simulink model "asyncSAR"  (R2024a)
settings: Solver=VariableStepAuto  StartTime=0.0  StopTime=0.0001844  RelTol=1e-3
model workspace (MAT data in the model file):
  Delay_106 = [1.91e-08 1.91e-08 1.91e-08]
  ENOB_106 = 9.63665810786
  FUNDF_106 = [9716803.44087 10062680.9808]
  FUNDX_106 = [81.3083483231 5.0894765013]
  IMODF_106 = [9396360.87497 10437767.0357]
  IMODX_106 = [6.9941846041 -2.14386455151]
  NoiseFloor_106 = -8.45635788485
  OIP3_106 = 63.5857886051
  SFDR_106 = 76.5977909113
  SINAD_106 = 59.7726818093
  SNR_106 = 59.7770481612
  THD_106 = -82.4847133329
  delay_106 = [1.91e-08 1.91e-08 1.91e-08]
libraries: msbAdcMeasurements x1, spsEdgeDetectorLib x1, dspsigops x1
settings Model: Creator=sjtu  LastModifiedBy=sjtu
settings DebuggingCC: SFUnexpectedBacktrackingDiag=warning

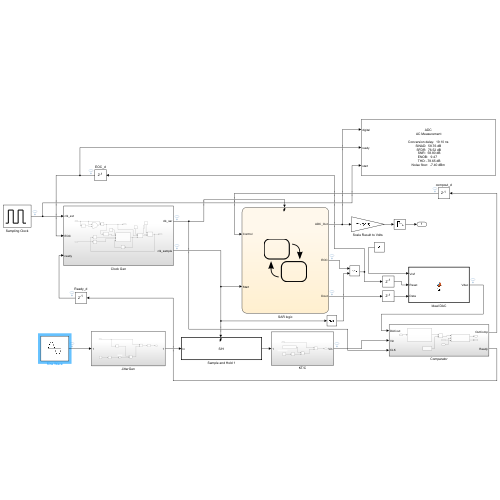
[thumbnail: Simulink's stored preview of the top-level diagram]
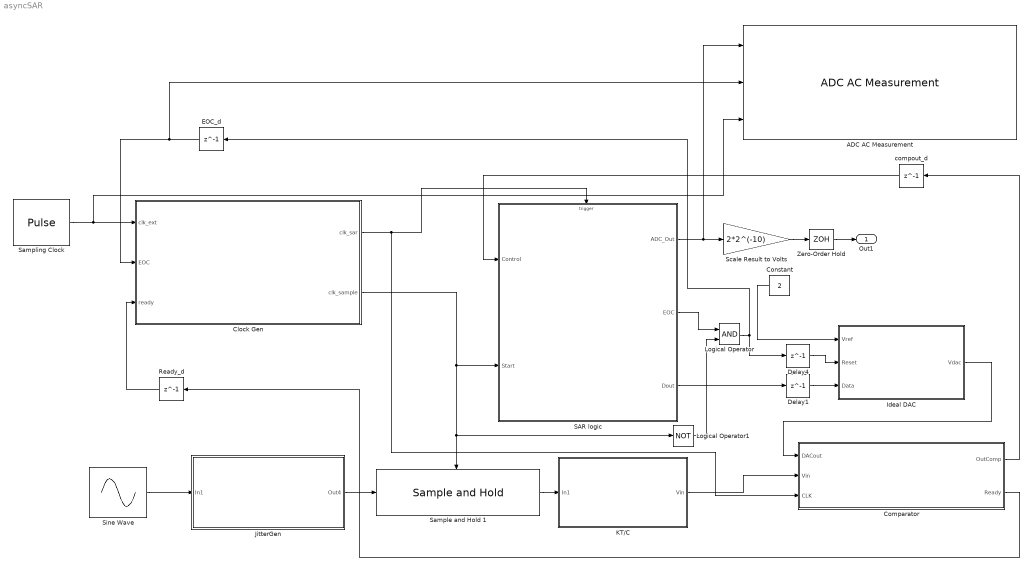
== system asyncSAR ==
  ADC AC Measurement : msbAdcMeasurements/ADC AC Measurement  DistortionMeasurement=Harmonic  InputFrequency=9.729e6  Method=Filter bank (slower, more precise, low leakage)  RBW=48828.125  AutoSetRBW=on  NBits=5  Frequency=5e7  HoldOffTime=0  OutputToWorkspace=off  VariableName=adc_ac_out  ShowSpectrum=off
  Clock Gen : Subsystem
  Comparator : Subsystem
  Constant : Constant  Value=2
  Delay1 : Delay  DelayLength=1  InitialCondition=0  SampleTime=1e-10
  Delay4 : Delay  DelayLength=1  InitialCondition=0  SampleTime=1e-10
  EOC_d : Delay  DelayLength=1  InitialCondition=0  SampleTime=1e-10
  Ideal DAC : MATLAB Function  TreatAsAtomicUnit=on
  JitterGen : Subsystem
  KT/C : Subsystem
  Logical Operator : Logic  AllPortsSameDT=off  OutDataTypeStr=boolean
  Logical Operator1 : Logic  Operator=NOT  AllPortsSameDT=off  OutDataTypeStr=boolean
  Ready_d : Delay  DelayLength=1  InitialCondition=0  SampleTime=1e-10
  SAR logic : Stateflow chart  TreatAsAtomicUnit=on
  Sample and Hold 1 : dspsigops/Sample and Hold  trig=Rising edge  initCond=0  latchinput=off
  Sampling Clock : DiscretePulseGenerator  PulseType=Time based  Period=1/(5e7)  PulseWidth=50  PhaseDelay=1e-9
  Scale Result to Volts : Gain  Gain=2*2^(-10)  ParamDataTypeStr=double  OutDataTypeStr=double
  Sine Wave : Sin  Frequency=2*pi*9.729e6  SampleTime=0
  Zero-Order Hold : ZeroOrderHold  SampleTime=-1
  compout_d : Delay  DelayLength=1  InitialCondition=0  SampleTime=1e-10
  Out1 : Outport
  wires:
  SAR logic/3(Dout) -> Delay1/1
  Delay1/1 -> Ideal DAC/3(Data)
  Zero-Order Hold/1 -> Out1/1
  Constant/1 -> Ideal DAC/1(Vref)
  Ideal DAC/1(Vdac) -> Comparator/1(DACout)
  SAR logic/1(ADC_Out) -> ADC AC Measurement/1, Scale Result to Volts/1
  JitterGen/1(Out4) -> Sample and Hold 1/1
  Scale Result to Volts/1 -> Zero-Order Hold/1
  Sample and Hold 1/1 -> KT/C/1(In1)
  KT/C/1(Vin) -> Comparator/2(Vin)
  Sine Wave/1 -> JitterGen/1(In1)
  Sampling Clock/1 -> ADC AC Measurement/3, Clock Gen/1(clk_ext)
  Comparator/2(Ready) -> Ready_d/1
  Ready_d/1 -> Clock Gen/3(ready)
  EOC_d/1 -> ADC AC Measurement/2, Clock Gen/2(EOC)
  Clock Gen/2(clk_sample) -> SAR logic/2(Start), Sample and Hold 1/Trigger, Logical Operator1/1
  Clock Gen/1(clk_sar) -> Comparator/3(CLK), SAR logic/Trigger
  Delay4/1 -> Ideal DAC/2(Reset)
  Logical Operator1/1 -> Logical Operator/2
  SAR logic/2(EOC) -> Logical Operator/1
  Logical Operator/1 -> EOC_d/1, Delay4/1
  Comparator/1(OutComp) -> compout_d/1
  compout_d/1 -> SAR logic/1(Control)

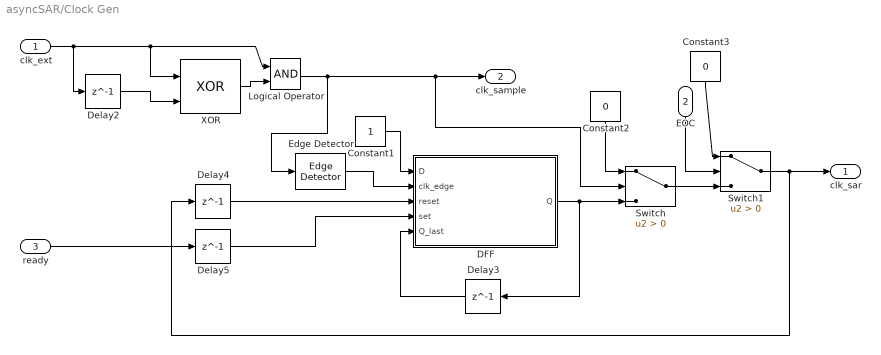
== system asyncSAR/Clock Gen ==
  clk_ext : Inport
  EOC : Inport  Port=2
  ready : Inport  Port=3
  Constant1 : Constant
  Constant2 : Constant  Value=0
  Constant3 : Constant  Value=0
  DFF : MATLAB Function  TreatAsAtomicUnit=on
  Delay2 : Delay  DelayLength=1  InitialCondition=0  SampleTime=2e-9
  Delay3 : Delay  DelayLength=1  InitialCondition=0  SampleTime=1e-10
  Delay4 : Delay  DelayLength=1  InitialCondition=0  SampleTime=4e-10
  Delay5 : Delay  DelayLength=1  InitialCondition=0  SampleTime=4e-10
  Edge Detector : spsEdgeDetectorLib/Edge Detector  model=Rising  ic=0  Ts=0
      settings: LibrarySourceBlock=sps_lib/Control/Edge Detector
  Logical Operator : Logic  AllPortsSameDT=off  OutDataTypeStr=boolean
  Switch : Switch  Criteria=u2 > Threshold  SaturateOnIntegerOverflow=off  InputSameDT=off
  Switch1 : Switch  Criteria=u2 > Threshold  SaturateOnIntegerOverflow=off  InputSameDT=off
  XOR : Logic  Operator=XOR  IconShape=distinctive  AllPortsSameDT=off  OutDataTypeStr=boolean
  clk_sar : Outport
  clk_sample : Outport  Port=2
  wires:
  Delay2/1 -> XOR/2
  clk_ext/1 -> Delay2/1, Logical Operator/1, XOR/1
  Switch/1 -> Switch1/3
  XOR/1 -> Logical Operator/2
  EOC/1 -> Switch1/2
  Logical Operator/1 -> Edge Detector/1, clk_sample/1, Switch/2
  DFF/1(Q) -> Switch/3, Delay3/1
  Constant3/1 -> Switch1/1
  Constant1/1 -> DFF/1(D)
  Delay5/1 -> DFF/4(set)
  Delay3/1 -> DFF/5(Q_last)
  Switch1/1 -> clk_sar/1, Delay4/1
  ready/1 -> Delay5/1
  Delay4/1 -> DFF/3(reset)
  Constant2/1 -> Switch/1
  Edge Detector/1 -> DFF/2(clk_edge)

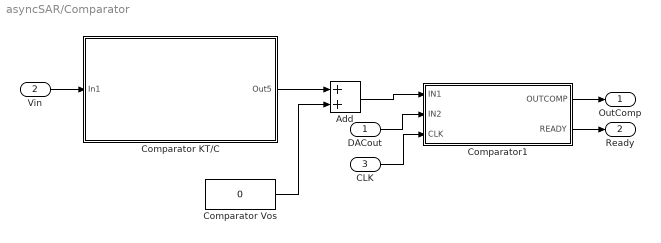
== system asyncSAR/Comparator ==
  DACout : Inport
  Vin : Inport  Port=2
  CLK : Inport  Port=3
  Add : Sum
  Comparator KT/C : Subsystem
  Comparator Vos : Constant  Value=0
  Comparator1 : MATLAB Function  TreatAsAtomicUnit=on
  OutComp : Outport
  Ready : Outport  Port=2
  wires:
  Comparator1/1(OUTCOMP) -> OutComp/1
  Vin/1 -> Comparator KT/C/1(In1)
  Comparator KT/C/1(Out5) -> Add/1
  Add/1 -> Comparator1/1(IN1)
  Comparator Vos/1 -> Add/2
  DACout/1 -> Comparator1/2(IN2)
  CLK/1 -> Comparator1/3(CLK)
  Comparator1/2(READY) -> Ready/1

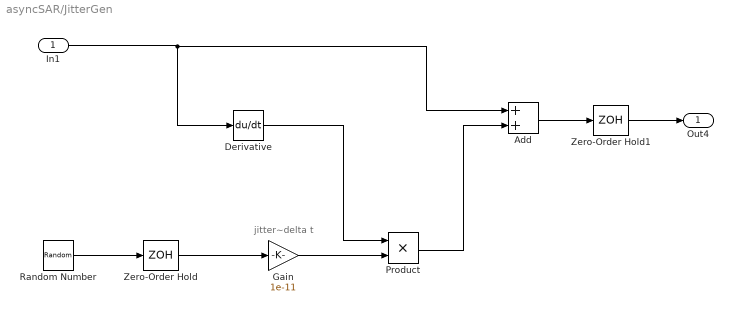
== system asyncSAR/JitterGen ==
  note: jitter~delta t
  In1 : Inport
  Add : Sum
  Derivative : Derivative
  Gain : Gain  Gain=1e-11
  Product : Product
  Random Number : RandomNumber  SampleTime=1e-9
  Zero-Order Hold : ZeroOrderHold  SampleTime=-1
  Zero-Order Hold1 : ZeroOrderHold  SampleTime=-1
  Out4 : Outport
  wires:
  Gain/1 -> Product/2
  Random Number/1 -> Zero-Order Hold/1
  Product/1 -> Add/2
  In1/1 -> Add/1, Derivative/1
  Zero-Order Hold/1 -> Gain/1
  Add/1 -> Zero-Order Hold1/1
  Derivative/1 -> Product/1
  Zero-Order Hold1/1 -> Out4/1

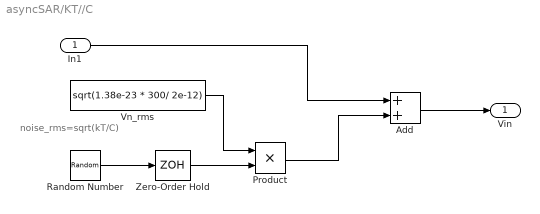
== system asyncSAR/KT//C ==
  note: noise_rms=sqrt(kT/C)
  In1 : Inport
  Add : Sum
  Product : Product
  Random Number : RandomNumber  SampleTime=1e-9
  Vn_rms : Constant  Value=sqrt(1.38e-23 * 300/ 2e-12)
  Zero-Order Hold : ZeroOrderHold  SampleTime=-1
  Vin : Outport
  wires:
  Vn_rms/1 -> Product/1
  In1/1 -> Add/1
  Random Number/1 -> Zero-Order Hold/1
  Zero-Order Hold/1 -> Product/2
  Add/1 -> Vin/1
  Product/1 -> Add/2

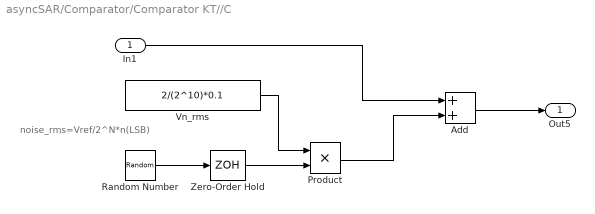
== system asyncSAR/Comparator/Comparator KT//C ==
  note: noise_rms=Vref/2^N*n(LSB)
  In1 : Inport
  Add : Sum
  Product : Product
  Random Number : RandomNumber  SampleTime=1e-9
  Vn_rms : Constant  Value=2/(2^10)*0.1
  Zero-Order Hold : ZeroOrderHold  SampleTime=-1
  Out5 : Outport
  wires:
  Vn_rms/1 -> Product/1
  In1/1 -> Add/1
  Random Number/1 -> Zero-Order Hold/1
  Zero-Order Hold/1 -> Product/2
  Add/1 -> Out5/1
  Product/1 -> Add/2

== matlab function asyncSAR/Ideal DAC ==
  data: Vref input; Reset input; Data input; Vdac output
function Vdac = fcn(Vref,Reset,Data)
if Reset==1
    Vdac=0;
else
    Vdac=double(Data)*Vref/(2^10);
end

== matlab function asyncSAR/Comparator/Comparator1 ==
  data: IN1 input; OUTCOMP output; IN2 input; CLK input; READY output
function [OUTCOMP,READY] = fcn(IN1,IN2,CLK)
if CLK==1
    READY=0;
else    
    READY=1;
end
if IN1>=IN2
        OUTCOMP=1;
else
        OUTCOMP=0;
end

== stateflow chart asyncSAR/SAR logic ==
  settings: executeAtInitialization=1
  state Idle_Done
    entry: Bit=9;
    EOC=1;
    ADC_Out=Dout;
  state Run
    entry: Dout=Dout+2^Bit;
  (default) -> Idle_Done
  Idle_Done -> Idle_Done [order 2] : [Start==1]{Dout=0;}
  (junction 26) -> Idle_Done [order 2] : [Bit==0]{EOC=1;}
  Idle_Done -> Run [order 1] : [Start==0]{Dout=-2^Bit;EOC=0;}
  (junction 26) -> Run [order 1] : [Bit>0]{Bit=Bit-1;}
  Run -> (junction 7) [order 2] : [Control==1]
  Run -> (junction 7) [order 1] : [Control==0]{Dout=Dout-2^Bit;}
  (junction 7) -> (junction 26)
  data: Control input; Start input; ADC_Out output int16; EOC output; Bit local double =9; Dout output int16
  events: clk input RISING_EDGE_EVENT

== matlab function asyncSAR/Clock Gen/DFF ==
  data: D input; Q output; clk_edge input; reset input; set input; Q_last input
function Q = fcn(D,clk_edge,reset,set,Q_last)

if (set==1)&&(reset==0)
    Q=1;
elseif (set==0)&&(reset==1)
    Q=0;
elseif (set==1)&&(reset==1)
    Q=Q_last;
else
    if clk_edge==1
        Q=D;
    else
        Q=Q_last;
    end
end
